simulink model "MLC_Kalman_Sim"  (R2019b)
settings: Solver=VariableStepAuto  StartTime=0.0  StopTime=20.0  RelTol=1e-3
values from neighbouring files (symbols this model uses):
  KF_sys = ss(A,B,C,D)    [MLC_Kalman.m]
undefined symbols (not defined in the file or in its folder): m_coeff
settings Model: Creator=idelafuentef  LastModifiedBy=idelafuentef

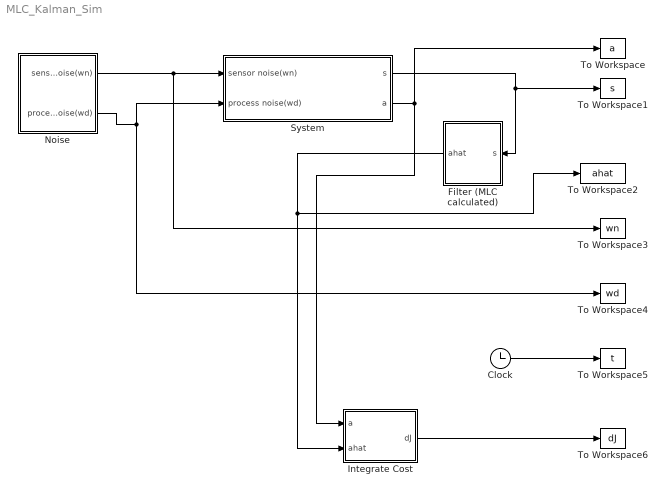
== system MLC_Kalman_Sim ==
  Clock : Clock
      settings: Decimation=20
  Filter (MLC calculated) : Subsystem
  Integrate Cost : Subsystem
  Noise : Subsystem
  System : Subsystem
  To Workspace : ToWorkspace  VariableName=a  SaveFormat=Timeseries  SampleTime=-1
  To Workspace1 : ToWorkspace  VariableName=s  SaveFormat=Timeseries  SampleTime=-1
  To Workspace2 : ToWorkspace  VariableName=ahat  SaveFormat=Timeseries  SampleTime=-1
  To Workspace3 : ToWorkspace  VariableName=wn  SaveFormat=Timeseries  SampleTime=-1
  To Workspace4 : ToWorkspace  VariableName=wd  SaveFormat=Timeseries  SampleTime=-1
  To Workspace5 : ToWorkspace  VariableName=t  SaveFormat=Timeseries  SampleTime=-1
  To Workspace6 : ToWorkspace  VariableName=dJ  SaveFormat=Timeseries  SampleTime=-1
  wires:
  Integrate Cost/1(dJ) -> To Workspace6/1
  Filter (MLC calculated)/1(ahat) -> To Workspace2/1, Integrate Cost/2(ahat)
  Noise/1(sensor noise(wn)) -> To Workspace3/1, System/1(sensor noise(wn))
  Noise/2(process noise(wd)) -> To Workspace4/1, System/2(process noise(wd))
  Clock/1 -> To Workspace5/1
  System/1(s) -> To Workspace1/1, Filter (MLC calculated)/1(s)
  System/2(a) -> Integrate Cost/1(a), To Workspace/1

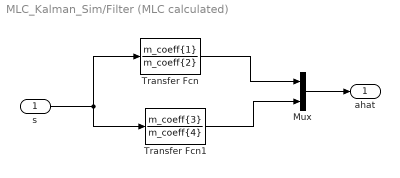
== system MLC_Kalman_Sim/Filter (MLC calculated) ==
  s : Inport
  Mux : Mux  Inputs=2
  Transfer Fcn : TransferFcn  Numerator=m_coeff{1}  Denominator=m_coeff{2}
  Transfer Fcn1 : TransferFcn  Numerator=m_coeff{3}  Denominator=m_coeff{4}
  ahat : Outport
  wires:
  s/1 -> Transfer Fcn1/1, Transfer Fcn/1
  Transfer Fcn/1 -> Mux/1
  Mux/1 -> ahat/1
  Transfer Fcn1/1 -> Mux/2

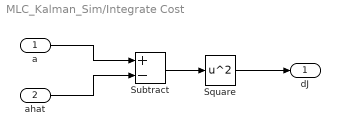
== system MLC_Kalman_Sim/Integrate Cost ==
  a : Inport
  ahat : Inport  Port=2
  Square : Math  Operator=square  SignedPower=off  SaturateOnIntegerOverflow=on
  Subtract : Sum  Inputs=+-
  dJ : Outport
  wires:
  Square/1 -> dJ/1
  Subtract/1 -> Square/1
  a/1 -> Subtract/1
  ahat/1 -> Subtract/2

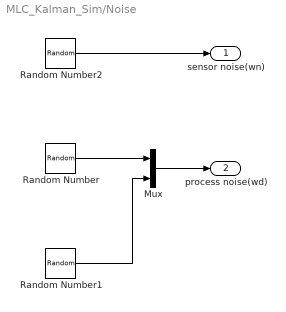
== system MLC_Kalman_Sim/Noise ==
  Mux : Mux  Inputs=2
  Random Number : RandomNumber  SampleTime=0.01
  Random Number1 : RandomNumber  Mean=1  SampleTime=0.01
  Random Number2 : RandomNumber  Variance=0.1  SampleTime=0.01
  sensor noise(wn) : Outport
  process noise(wd) : Outport  Port=2  PortDimensions=2
  wires:
  Random Number2/1 -> sensor noise(wn)/1
  Random Number/1 -> Mux/1
  Random Number1/1 -> Mux/2
  Mux/1 -> process noise(wd)/1

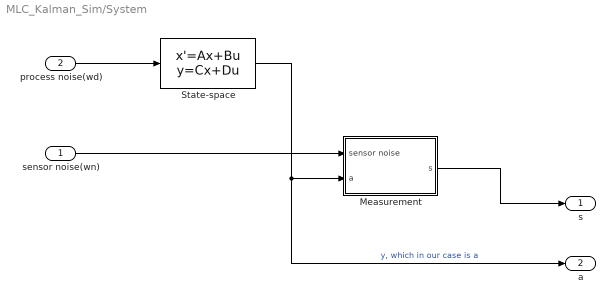
== system MLC_Kalman_Sim/System ==
  sensor noise(wn) : Inport
  process noise(wd) : Inport  Port=2
  Measurement : Subsystem
  State-space : StateSpace  A=KF_sys.A  B=KF_sys.B  C=KF_sys.C  D=KF_sys.D  InitialCondition=[1 0]
  s : Outport
  a : Outport  Port=2
  wires:
  State-space/1 -> Measurement/2(a), a/1  "y, which in our case is a"
  Measurement/1(s) -> s/1
  sensor noise(wn)/1 -> Measurement/1(sensor noise)
  process noise(wd)/1 -> State-space/1

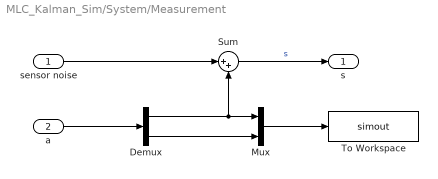
== system MLC_Kalman_Sim/System/Measurement ==
  sensor noise : Inport
  a : Inport  Port=2
  Demux : Demux  Outputs=2
  Mux : Mux  Inputs=2
  Sum : Sum  Inputs=|++
  To Workspace : ToWorkspace  VariableName=simout  SaveFormat=Timeseries  SampleTime=-1
  s : Outport
  wires:
  Sum/1 -> s/1  "s"
  Demux/1 -> Mux/1, Sum/2
  sensor noise/1 -> Sum/1
  a/1 -> Demux/1
  Demux/2 -> Mux/2
  Mux/1 -> To Workspace/1
